simulink model "LQG_test"  (R2015a)
settings: Solver=ode5  StartTime=0.0  StopTime=160  FixedStep=1e-4  RelTol=1e-3
values from neighbouring files (symbols this model uses):
  Af = [-15.9802071238 -2566.97948561 -96.8709621573 -60.7443875975 -54.1893771527 41.3534774927 -111.758131839 -5.18957577709 4.71062280365 61.452788526 0.0297969919136 0.177289731224 ... (144 elements, 12x12)]    [identified_t1_full.mat]
  Ak = [-672.634870495 -2626.58972998 -46.1193303275 25.5793500122 108.891317034 -102.718752792 -245.794654799 -577.315326704 39.8827087547 153.58157137 60.36854216 -207.81122515 ... (144 elements, 12x12)]    [controller.mat]    (also in main_matlab_single_step.m = rlqg.A)
  Bf = [-0.242989780525 -0.0299322746251 0.321554597542 0.228133316924 0.286172349315 -0.305996080434 -0.00624937622709 0.299905571178 0.0491887335661 0.146540635678 -0.0583489322764 0.229737532171 ... (24 elements, 12x2)]    [identified_t1_full.mat]
  Bk = [0.204306341627 1.11161335273 -0.324978673641 2.85402340631 -4.5813117605 2.97328839236 -0.174709893359 1.31662160979 2.94898293865 13.5567055967 -0.791381118401 0.0552385579013]    [controller.mat]    (also in main_matlab_single_step.m = rlqg.B)
  Cf = [11.6526185223 -2.27862995386 -17.2646212697 -3.07480298339 -1.84306279106 6.13326135217 -7.61687548654 -1.01458329844 1.12240644674 6.24617551809 15.4271955414 -17.0295297306]    [identified_t1_full.mat]
  Ck = [534.788956442 909.016401092 107.069958755 -410.092366717 -1097.26369634 478.53061829 -894.210554118 460.341899649 -450.064931583 371.993181033 532.787728171 55.8162878584 ... (24 elements, 2x12)]    [controller.mat]    (also in main_matlab_single_step.m = rlqg.C)
  Dk = [0 0]    [controller.mat]    (also in main_matlab_single_step.m = rlqg.D)
  Hf = [-0.00603819148621 -0.0121645329261 0.00178372873077 -0.020497816306 0.0668191856228 0.0461443111066 0.00197372154204 -0.00747704137343 -0.135635344699 -0.102773865384 0.0647006981549 0.0468916096625]    [identified_t1_full.mat]
libraries: simulink x1
settings Model: Creator=p4wp4w  LastModifiedBy=Ablah

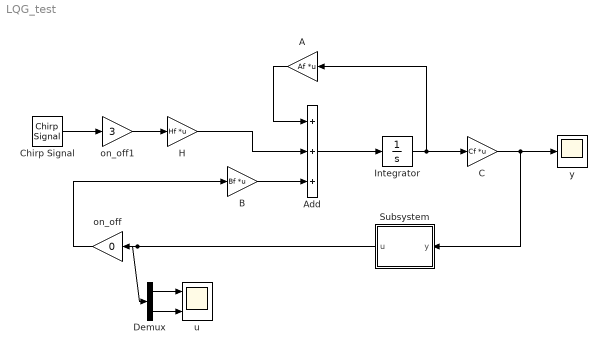
== system LQG_test ==
  A : Gain  Gain=Af  Multiplication=Matrix(K*u)
  Add : Sum  Inputs=+++
  B : Gain  Gain=Bf  Multiplication=Matrix(K*u)
  C : Gain  Gain=Cf  Multiplication=Matrix(K*u)
  Chirp Signal : simulink/Sources/Chirp Signal  f1=0.1  T=80  f2=800
  Demux : Demux  Outputs=2
  H : Gain  Gain=Hf  Multiplication=Matrix(K*u)
  Integrator : Integrator
  Subsystem : Subsystem
  on_off : Gain  Gain=0
  on_off1 : Gain  Gain=3
  u : Scope  NumInputPorts=2
      settings: YMin=-5~-5  YMax=5~5
  y : Scope
      settings: YMin=-0.03  YMax=0.03
  wires:
  Add/1 -> Integrator/1
  A/1 -> Add/1
  B/1 -> Add/3
  Integrator/1 -> C/1, A/1
  H/1 -> Add/2
  Chirp Signal/1 -> on_off1/1
  on_off/1 -> B/1
  Demux/1 -> u/1
  Demux/2 -> u/2
  C/1 -> Subsystem/1(y), y/1
  Subsystem/1("u ") -> Demux/1, on_off/1
  on_off1/1 -> H/1

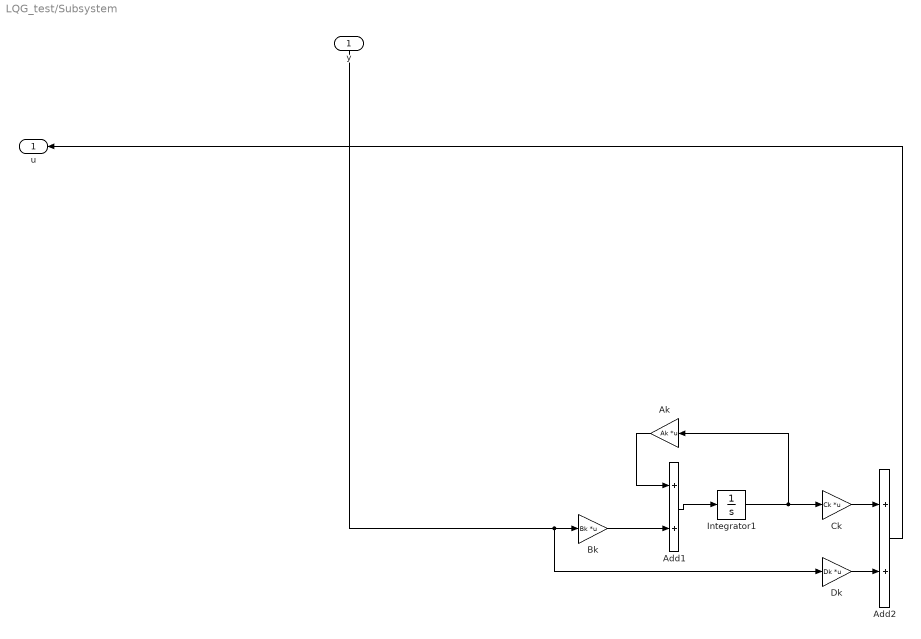
== system LQG_test/Subsystem ==
  y : Inport
  Add1 : Sum
  Add2 : Sum
  Ak : Gain  Gain=Ak  Multiplication=Matrix(K*u)
  Bk : Gain  Gain=Bk  Multiplication=Matrix(K*u)
  Ck : Gain  Gain=Ck  Multiplication=Matrix(K*u)
  Dk : Gain  Gain=Dk  Multiplication=Matrix(K*u)
  Integrator1 : Integrator
  "u " : Outport
  wires:
  y/1 -> Bk/1, Dk/1
  Add2/1 -> "u "/1
  Bk/1 -> Add1/2
  Ak/1 -> Add1/1
  Add1/1 -> Integrator1/1
  Dk/1 -> Add2/2
  Integrator1/1 -> Ck/1, Ak/1
  Ck/1 -> Add2/1
